simulink model "SwitchFilter"  (R2018b)
settings: Solver=FixedStepAuto  StartTime=0.0  StopTime=10.0  FixedStep=0.02  RelTol=1e-3
undefined symbols (not defined in the file): sigbuilder_block
libraries: simulink x1
settings Model: Creator=novauto  LastModifiedBy=novauto

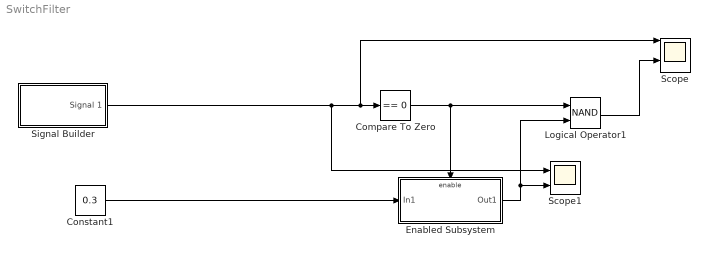
== system SwitchFilter ==
  Compare To Zero : simulink/Logic and Bit Operations/Compare To Zero  relop===  OutDataTypeStr=boolean
  Constant1 : Constant  Value=0.3
  Enabled Subsystem : Subsystem  TreatAsAtomicUnit=on
  Logical Operator1 : Logic  Operator=NAND  AllPortsSameDT=off  OutDataTypeStr=boolean
  Scope : Scope  NumInputPorts=4
  Scope1 : Scope  NumInputPorts=2
  Signal Builder : Subsystem  Tag=STV Subsys  LoadFcn=sigbuilder_block('load');  StartFcn=sigbuilder_block('start');  StopFcn=sigbuilder_block('stop');  ClipboardFcn=sigbuilder_block('clipboard');  mask(Sigbuilder block){tuvar=[0:10]}
      mask help: Simulink:masks:SigbuilderBlock_MD
      mask init:
      | if ~strcmp(get_param(bdroot(gcbh),'SimulationStatus'),'stopped') tuvar = sigbuilder_block('maskInit'); end
      settings: CopyFcn=sigbuilder_block('copy');  DeleteFcn=sigbuilder_block('delete');  ModelCloseFcn=sigbuilder_block('modelClose');  PreSaveFcn=sigbuilder_block('preSave');  PauseFcn=sigbuilder_block('pause');  ContinueFcn=sigbuilder_block('continue');  NameChangeFcn=sigbuilder_block('namechange');  OpenFcn=sigbuilder_block('open',[437.25 199.5 550.5 399.75 ]);  CloseFcn=sigbuilder_block('close');
      mask Display: plot(0, 0, 100, 100,[2, 2, 32, 32, 2], [68, 8, 8, 68, 68],[32, 2], [38, 38], [32, 19, 2],[53, 60, 44], [32, 17, 17, 2],[16, 16, 31, 31]);txt = getActiveGroup(gcbh);text(2, 100, txt,'verticalAlignment', 'top');
  wires:
  Signal Builder/1(Signal 1) -> Scope1/1, Scope/1, Compare To Zero/1
  Compare To Zero/1 -> Logical Operator1/1, Enabled Subsystem/Enable
  Enabled Subsystem/1(Out1) -> Scope1/2, Logical Operator1/2
  Logical Operator1/1 -> Scope/3
  Constant1/1 -> Enabled Subsystem/1(In1)

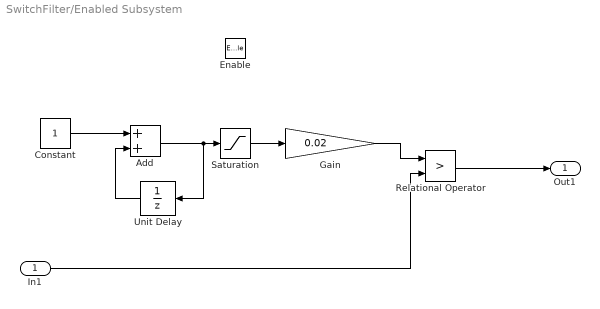
== system SwitchFilter/Enabled Subsystem ==
  In1 : Inport
  Enable : EnablePort  StatesWhenEnabling=reset
  Add : Sum  SaturateOnIntegerOverflow=on
  Constant : Constant
  Gain : Gain  Gain=0.02
  Relational Operator : RelationalOperator  Operator=>  OutDataTypeStr=boolean  RndMeth=Simplest
  Saturation : Saturate  UpperLimit=50000  LowerLimit=0
  Unit Delay : UnitDelay  SampleTime=-1
  Out1 : Outport  OutputWhenDisabled=reset  InitialOutput=1
  wires:
  Constant/1 -> Add/1
  Add/1 -> Unit Delay/1, Saturation/1
  Gain/1 -> Relational Operator/1
  Relational Operator/1 -> Out1/1
  Unit Delay/1 -> Add/2
  In1/1 -> Relational Operator/2
  Saturation/1 -> Gain/1

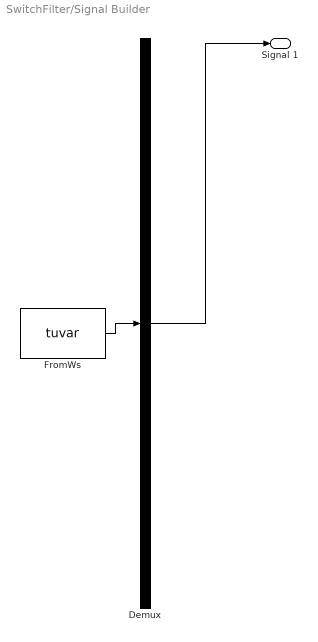
== system SwitchFilter/Signal Builder ==
  Demux : Demux  Tag=STV Demux  Outputs=1
  FromWs : FromWorkspace  Tag=STV FromWs  VariableName=tuvar  SampleTime=0
      SigBuilderData=|
      | common.afterFinalStr = 'Extrapolate'
      | common.sampleTime = 0
      | dataSet.timeRange = [0 10]
      | dataSet.name = 'Group 1'
      | sbobj.Groups.Name = 'Group 1'
      | sbobj.Groups.Signals.Name = 'Signal 1'
      | sbobj.Groups.Signals.XData = [0 1.02 1.02 1.2 1.2 1.4 1.4 1.6 1.6 1.8 1.8 2 2 3.62 3.62 4.22 4.22 4.58 4.58 5.1 5.1 5.48 5.48 6 6 10]
      | sbobj.Groups.Signals.YData = [0 0 1 1 0 0 1 1 0 0 1 1 0 0 1 1 0 0 1 1 0 0 1 1 0 0]
  Signal 1 : Outport  Tag=STV Outport
  wires:
  Demux/1 -> Signal 1/1
  FromWs/1 -> Demux/1
